simulink subsystem "Fuel_economy"  (R2020b)
settings: Solver=VariableStepAuto  StartTime=0.0  StopTime=10.0  RelTol=1e-3
settings Model: Creator=galli  LastModifiedBy=galli

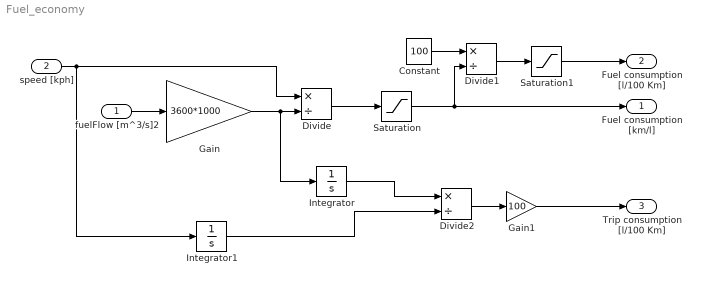
== system Fuel_economy ==
  fuelFlow [m^3/s]2 : Inport
  speed [kph] : Inport  Port=2
  Constant : Constant  Value=100
  Divide : Product  Inputs=*/
  Divide1 : Product  Inputs=*/
  Divide2 : Product  Inputs=*/
  Gain : Gain  Gain=3600*1000
  Gain1 : Gain  Gain=100
  Integrator : Integrator
  Integrator1 : Integrator
  Saturation : Saturate  UpperLimit=100  LowerLimit=0
  Saturation1 : Saturate  UpperLimit=25  LowerLimit=0
  Fuel consumption [km/l] : Outport
  Fuel consumption [l/100 Km] : Outport  Port=2
  Trip consumption [l/100 Km] : Outport  Port=3
  wires:
  Divide2/1 -> Gain1/1
  Integrator/1 -> Divide2/1
  Gain/1 -> Integrator/1, Divide/2
  Saturation1/1 -> Fuel consumption [l/100 Km]/1
  Integrator1/1 -> Divide2/2
  Divide1/1 -> Saturation1/1
  fuelFlow [m^3/s]2/1 -> Gain/1
  Divide/1 -> Saturation/1
  speed [kph]/1 -> Integrator1/1, Divide/1
  Gain1/1 -> Trip consumption [l/100 Km]/1
  Saturation/1 -> Divide1/2, Fuel consumption [km/l]/1
  Constant/1 -> Divide1/1
